simulink library "inp"  (R2021b)
settings: Solver=VariableStepAuto  StartTime=0.0  StopTime=10.0  RelTol=1e-3
undefined symbols (not defined in the file): C_TASK_5MS_S, FALSE, KINP_AcoreReadyToSlp_flg_ovrdflg, KINP_AcoreReadyToSlp_flg_ovrdval, KINP_AllowMovThd_OTA_enum_ovrdflg, KINP_AllowMovThd_OTA_enum_ovrdval, KINP_APSAngleTarget_Deg_ovrdflg, KINP_APSAngleTarget_Deg_ovrdval, KINP_APSDecReq_mps2_ovrdflg, KINP_APSDecReq_mps2_ovrdval, KINP_APSDecReqA_flg_ovrdflg, KINP_APSDecReqA_flg_ovrdval, KINP_APSDFLL_cm_ovrdflg, KINP_APSDFLL_cm_ovrdval, KINP_APSDFLR_cm_ovrdflg, KINP_APSDFLR_cm_ovrdval, KINP_APSDRLL_cm_ovrdflg, KINP_APSDRLL_cm_ovrdval, KINP_APSDRLR_cm_ovrdflg, KINP_APSDRLR_cm_ovrdval, KINP_APSExitCondition_enum_ovrdflg, KINP_APSExitCondition_enum_ovrdval, KINP_APSHWVer_enum_ovrdflg, KINP_APSHWVer_enum_ovrdval, KINP_APSProgressPCT_pct_ovrdflg, KINP_APSProgressPCT_pct_ovrdval, KINP_APSReq_enum_ovrdflg, KINP_APSReq_enum_ovrdval, KINP_APSRQDisplay_enum_ovrdflg, KINP_APSRQDisplay_enum_ovrdval, KINP_APSRqEPASCtrl_flg_ovrdflg, KINP_APSRqEPASCtrl_flg_ovrdval, KINP_APSShiftPosnReq_enum_ovrdval, KINP_APSShiftPosnReq_enum_ovrflg, KINP_APSSpeedCMD_kph_ovrdval, KINP_APSSpeedCMD_kph_ovrflg, KINP_APSStaSystem_enum_ovrdflg, KINP_APSStaSystem_enum_ovrdval, KINP_APSSWVer_enum_ovrdflg, KINP_APSSWVer_enum_ovrdval, KINP_APSVMCReqA_flg_ovrdval, KINP_APSVMCReqA_flg_ovrflg, KINP_APSVRqEPASCtrl_flg_ovrdflg, KINP_APSVRqEPASCtrl_flg_ovrdval, KINP_AuxBattVolmV_mV_ovrdflg, KINP_AuxBattVolmV_mV_ovrdval, KINP_CAASSta_enum_ovrdflg, KINP_CAASSta_enum_ovrdval, KINP_CAASVMCReqA_flg_ovrdval, KINP_CAASVMCReqA_flg_ovrflg, KINP_Chime_enum_ovrdflg, KINP_Chime_enum_ovrdval, KINP_ClearDTCcmd_flg_ovrdflg, KINP_ClearDTCcmd_flg_ovrdval, KINP_EvccAplusPwrUpReq_flg_ovrdflg, KINP_EvccAplusPwrUpReq_flg_ovrdval, KINP_LFID_raw_ovrdval, KINP_LFID_raw_ovrflg, KINP_LRID_raw_ovrdval, KINP_MemOffsetAccX_raw16_ovrdflg ... (+118)
libraries: FVT_lib x595, hcu_lib x1
(part 7 of 27)

== system inp/INP/CAN4/CreateBus ==
  inp_CanValid_bus : Inport
  inp_Hal_bus : Inport  Port=2
  UnitConverter_{1..14,24,26,31,34,38..40,44..49,60..61,63..64,97..99,102,108} (36 alike) : DataTypeConversion  OutDataTypeStr=boolean
  UnitConverter_{42..43,50..53,55..59,62,66,69,71,73,75,77,79,81,83,85,87,89..90,92..93,100..101,103..104,106,112,114,121,123,125,127,129,131,133,135,141} (43 alike) : DataTypeConversion  OutDataTypeStr=single
  UnitConverter_{15..23,25,30,32..33,35..37,41,54,65,67..68,70,72,74,76,78,80,82,84,86,88,91,94..96,105,107,109..111,113,115..120,122,124,126,128,130,132,134,136..140,142} (60 alike) : DataTypeConversion  OutDataTypeStr=uint8
  UnitConverter_27 : DataTypeConversion  OutDataTypeStr=uint64
  UnitConverter_28 : DataTypeConversion  OutDataTypeStr=uint64
  UnitConverter_29 : DataTypeConversion  OutDataTypeStr=uint64
  bus_creator : BusCreator  Inputs=142
  bus_selector : BusSelector  OutputSignals=VINP_CANMsgValidDKC1_flg,VINP_CANMsgValidDKC2_flg,VINP_CANMsgValidGWZDRPTG1_flg,VINP_CANMsgValidGWZoneDR1_flg,VINP_CANMsgValidGWZoneDR2_flg,VINP_CANMsgValidGWZoneDR3_flg,VINP_CANMsgValidGWZoneDR4_flg,VINP_CANMsgValidGWZoneDR6_flg,VINP_CANMsgValidGWZoneFR1_flg,VINP_CANMsgValidGWZoneFR2_flg,VINP_CANMsgValidZoneDrSCP_flg,VINP_CANMsgValidZoneDrTHCM_flg,VINP_CANMsgValidZoneDrVCU_flg,VINP_CANMsgValidZoneFrTHCM_flg
  bus_selector_1 : BusSelector  OutputSignals=VINP_DKCReVehData_enum,VINP_DKCRemotePW_enum,VINP_PCommandToBCM_enum,VINP_PCommandToPTG_enum,VINP_PDKeyAreaLockUnlock_enum,VINP_PDKeyAreaPS_enum,VINP_PDKeyAreaPTG_enum,VINP_PDKeyWelcome_enum,VINP_PDkeyShowIVI_enum,VINP_PKeyMiss_flg,VINP_PKeyMode_enum,VINP_PUIDLowPower_flg,VINP_EncryptionDATA063_enum,VINP_EncryptionDATA64127_enum,VINP_RandomNumberX_enum,VINP_PTGRDILSta_enum,VINP_CSWDimSw_flg,VINP_CSWFWasSwSta_enum,VINP_CSWFWipSwSta_enum,VINP_CSWPassSWSta_flg,VINP_CSWRWasSWSta_enum,VINP_CSWRWipIntSwSta_enum,VINP_CSWTurnSwSta_enum,VINP_DrLockSta_flg,VINP_MIRRORFOLDSW_flg,VINP_RLSLampSta_flg,VINP_RLSRainSnrWiperCmd_enum,VINP_RLTurnLampC_mA,VINP_RRTurnLampC_mA,VINP_RWiperAS_flg,VINP_RWiperProtection_flg,VINP_SWCCANCELSta_flg,VINP_SWCResUpSta_flg,VINP_SWCSetdownSta_flg,VINP_SWCmodeSta_flg,VINP_LDrvValWdwOpened_pct,VINP_LPasValWdwOpened_pct,VINP_LRLDValWdwOpened_pct,VINP_LRRDValWdwOpened_pct,VINP_PTGInnerSW2_enum,VINP_FrntPTCRearLeActHeatPwr_W,VINP_FrntPTCRearRiActHeatPwr_W,VINP_FrntPTCRiActHeatPwr_W,VINP_FLTurnLampC_mA,VINP_FRTurnLampC_mA,VINP_FWiperAS_flg,VINP_FWiperProtection_flg,VINP_COMPStatorSpd_rpm,VINP_CompProEN_flg,VINP_DrSCPSysErrLmp_flg,VINP_RegenMode_enum,VINP_SetSpd_kph,VINP_ZoneSpdCtrlMode_enum,VINP_BlowerErr_enum,VINP_SolarL_W,VINP_SolarLErr_enum,VINP_SolarR_W,VINP_SolarRErr_enum,VINP_TFaceL_C,VINP_TFaceLErr_enum,VINP_TFaceR_C,VINP_TFaceRErr_enum,VINP_TFaceRr_C,VINP_TFaceRrErr_enum,VINP_TFootL_C,VINP_TFootLErr_enum,VINP_TFootR_C,VINP_TFootRErr_enum,VINP_TFootRr_C,VINP_TFootRrErr_enum,VINP_Tevap_C,VINP_TevapErr_enum,VINP_Tincar_C,VINP_TincarErr_enum,VINP_DrAuBoxPwrN1Curr_A,VINP_DrAuBoxPwrN2Curr_A,VINP_DrColumnSWFault_enum,VINP_DrCtrlBDVolt_V,VINP_DrCtrlTemp_C,VINP_DrEOBDFault_enum,VINP_DrIVIFault_enum,VINP_DrInfoFault_enum,VINP_DrPMMLVOutPErrLmp_flg,VINP_DrPMMLimpHomeActReq_flg,VINP_DrPMMSysErrLmp_flg,VINP_DrPowerTemp1_C,VINP_DrPowerTemp2_C,VINP_DrPwrInformationSta_flg,VINP_DrPwrONA1Curr_A,VINP_DrPwrONA2Curr_A,VINP_DrPwrSta_enum,VINP_DrPwrStdbyACurr_A,VINP_DrPwrWindowECUFault_enum,VINP_DrStdAErrSta_flg,VINP_DrTHCMFault_enum,VINP_ZoneDrMalfunLevel_enum,VINP_AGSErr_enum,VINP_BatInTemp_C,VINP_BatInTempErr_enum,VINP_BatOutTemp_C,VINP_COMPErr_enum,VINP_EACProtectEnable_enum,VINP_EWP3Err_enum,VINP_EXV1Err_enum,VINP_EXV2Err_enum,VINP_FanErr_enum,VINP_MotorInTemp_C,VINP_MotorInTempErr_enum,VINP_MotorOutTemp_C,VINP_MotorOutTempErr_enum,VINP_PTHighP_KPa,VINP_PTHighPErr_enum,VINP_PTHighTact_C,VINP_PTHighTactErr_enum,VINP_PTLowP1_KPa,VINP_PTLowP1Err_enum,VINP_PTLowP2_KPa,VINP_PTLowP2Err_enum,VINP_PTLowT1_C,VINP_PTLowT1Err_enum,VINP_PTLowT2_C,VINP_PTLowT2Err_enum,VINP_SOTXVErr_enum,VINP_SOV1Err_enum,VINP_SOV2Err_enum,VINP_SOV3Err_enum,VINP_Tamb_C,VINP_TambErr_enum
  BINP_outputs : Outport
  wires:
  inp_CanValid_bus/1 -> [inp_CanValid_bus]
  inp_Hal_bus/1 -> [inp_Hal_bus]
  bus_selector/1 -> UnitConverter_1/1  "<VINP_CANMsgValidDKC1_flg>"
  UnitConverter_1/1 -> bus_creator/1  "VINP_CANMsgValidDKC1_flg"
  bus_selector/2 -> UnitConverter_2/1  "<VINP_CANMsgValidDKC2_flg>"
  UnitConverter_2/1 -> bus_creator/2  "VINP_CANMsgValidDKC2_flg"
  bus_selector/3 -> UnitConverter_3/1  "<VINP_CANMsgValidGWZDRPTG1_flg>"
  UnitConverter_3/1 -> bus_creator/3  "VINP_CANMsgValidGWZDRPTG1_flg"
  bus_selector/4 -> UnitConverter_4/1  "<VINP_CANMsgValidGWZoneDR1_flg>"
  UnitConverter_4/1 -> bus_creator/4  "VINP_CANMsgValidGWZoneDR1_flg"
  bus_selector/5 -> UnitConverter_5/1  "<VINP_CANMsgValidGWZoneDR2_flg>"
  UnitConverter_5/1 -> bus_creator/5  "VINP_CANMsgValidGWZoneDR2_flg"
  bus_selector/6 -> UnitConverter_6/1  "<VINP_CANMsgValidGWZoneDR3_flg>"
  UnitConverter_6/1 -> bus_creator/6  "VINP_CANMsgValidGWZoneDR3_flg"
  bus_selector/7 -> UnitConverter_7/1  "<VINP_CANMsgValidGWZoneDR4_flg>"
  UnitConverter_7/1 -> bus_creator/7  "VINP_CANMsgValidGWZoneDR4_flg"
  bus_selector/8 -> UnitConverter_8/1  "<VINP_CANMsgValidGWZoneDR6_flg>"
  UnitConverter_8/1 -> bus_creator/8  "VINP_CANMsgValidGWZoneDR6_flg"
  bus_selector/9 -> UnitConverter_9/1  "<VINP_CANMsgValidGWZoneFR1_flg>"
  UnitConverter_9/1 -> bus_creator/9  "VINP_CANMsgValidGWZoneFR1_flg"
  bus_selector/10 -> UnitConverter_10/1  "<VINP_CANMsgValidGWZoneFR2_flg>"
  UnitConverter_10/1 -> bus_creator/10  "VINP_CANMsgValidGWZoneFR2_flg"
  bus_selector/11 -> UnitConverter_11/1  "<VINP_CANMsgValidZoneDrSCP_flg>"
  UnitConverter_11/1 -> bus_creator/11  "VINP_CANMsgValidZoneDrSCP_flg"
  bus_selector/12 -> UnitConverter_12/1  "<VINP_CANMsgValidZoneDrTHCM_flg>"
  UnitConverter_12/1 -> bus_creator/12  "VINP_CANMsgValidZoneDrTHCM_flg"
  bus_selector/13 -> UnitConverter_13/1  "<VINP_CANMsgValidZoneDrVCU_flg>"
  UnitConverter_13/1 -> bus_creator/13  "VINP_CANMsgValidZoneDrVCU_flg"
  bus_selector/14 -> UnitConverter_14/1  "<VINP_CANMsgValidZoneFrTHCM_flg>"
  UnitConverter_14/1 -> bus_creator/14  "VINP_CANMsgValidZoneFrTHCM_flg"
  bus_selector_1/1 -> UnitConverter_15/1  "<VINP_DKCReVehData_enum>"
  UnitConverter_15/1 -> bus_creator/15  "VINP_DKCReVehData_enum"
  bus_selector_1/2 -> UnitConverter_16/1  "<VINP_DKCRemotePW_enum>"
  UnitConverter_16/1 -> bus_creator/16  "VINP_DKCRemotePW_enum"
  bus_selector_1/3 -> UnitConverter_17/1  "<VINP_PCommandToBCM_enum>"
  UnitConverter_17/1 -> bus_creator/17  "VINP_PCommandToBCM_enum"
  bus_selector_1/4 -> UnitConverter_18/1  "<VINP_PCommandToPTG_enum>"
  UnitConverter_18/1 -> bus_creator/18  "VINP_PCommandToPTG_enum"
  bus_selector_1/5 -> UnitConverter_19/1  "<VINP_PDKeyAreaLockUnlock_enum>"
  UnitConverter_19/1 -> bus_creator/19  "VINP_PDKeyAreaLockUnlock_enum"
  bus_selector_1/6 -> UnitConverter_20/1  "<VINP_PDKeyAreaPS_enum>"
  UnitConverter_20/1 -> bus_creator/20  "VINP_PDKeyAreaPS_enum"
  bus_selector_1/7 -> UnitConverter_21/1  "<VINP_PDKeyAreaPTG_enum>"
  UnitConverter_21/1 -> bus_creator/21  "VINP_PDKeyAreaPTG_enum"
  bus_selector_1/8 -> UnitConverter_22/1  "<VINP_PDKeyWelcome_enum>"
  UnitConverter_22/1 -> bus_creator/22  "VINP_PDKeyWelcome_enum"
  bus_selector_1/9 -> UnitConverter_23/1  "<VINP_PDkeyShowIVI_enum>"
  UnitConverter_23/1 -> bus_creator/23  "VINP_PDkeyShowIVI_enum"
  bus_selector_1/10 -> UnitConverter_24/1  "<VINP_PKeyMiss_flg>"
  UnitConverter_24/1 -> bus_creator/24  "VINP_PKeyMiss_flg"
  bus_selector_1/11 -> UnitConverter_25/1  "<VINP_PKeyMode_enum>"
  UnitConverter_25/1 -> bus_creator/25  "VINP_PKeyMode_enum"
  bus_selector_1/12 -> UnitConverter_26/1  "<VINP_PUIDLowPower_flg>"
  UnitConverter_26/1 -> bus_creator/26  "VINP_PUIDLowPower_flg"
  bus_selector_1/13 -> UnitConverter_27/1  "<VINP_EncryptionDATA063_enum>"
  UnitConverter_27/1 -> bus_creator/27  "VINP_EncryptionDATA063_enum"
  bus_selector_1/14 -> UnitConverter_28/1  "<VINP_EncryptionDATA64127_enum>"
  UnitConverter_28/1 -> bus_creator/28  "VINP_EncryptionDATA64127_enum"
  bus_selector_1/15 -> UnitConverter_29/1  "<VINP_RandomNumberX_enum>"
  UnitConverter_29/1 -> bus_creator/29  "VINP_RandomNumberX_enum"
  bus_selector_1/16 -> UnitConverter_30/1  "<VINP_PTGRDILSta_enum>"
  UnitConverter_30/1 -> bus_creator/30  "VINP_PTGRDILSta_enum"
  bus_selector_1/17 -> UnitConverter_31/1  "<VINP_CSWDimSw_flg>"
  UnitConverter_31/1 -> bus_creator/31  "VINP_CSWDimSw_flg"
  bus_selector_1/18 -> UnitConverter_32/1  "<VINP_CSWFWasSwSta_enum>"
  UnitConverter_32/1 -> bus_creator/32  "VINP_CSWFWasSwSta_enum"
  bus_selector_1/19 -> UnitConverter_33/1  "<VINP_CSWFWipSwSta_enum>"
  UnitConverter_33/1 -> bus_creator/33  "VINP_CSWFWipSwSta_enum"
  bus_selector_1/20 -> UnitConverter_34/1  "<VINP_CSWPassSWSta_flg>"
  UnitConverter_34/1 -> bus_creator/34  "VINP_CSWPassSWSta_flg"
  bus_selector_1/21 -> UnitConverter_35/1  "<VINP_CSWRWasSWSta_enum>"
  UnitConverter_35/1 -> bus_creator/35  "VINP_CSWRWasSWSta_enum"
  bus_selector_1/22 -> UnitConverter_36/1  "<VINP_CSWRWipIntSwSta_enum>"
  UnitConverter_36/1 -> bus_creator/36  "VINP_CSWRWipIntSwSta_enum"
  bus_selector_1/23 -> UnitConverter_37/1  "<VINP_CSWTurnSwSta_enum>"
  UnitConverter_37/1 -> bus_creator/37  "VINP_CSWTurnSwSta_enum"
  bus_selector_1/24 -> UnitConverter_38/1  "<VINP_DrLockSta_flg>"
  UnitConverter_38/1 -> bus_creator/38  "VINP_DrLockSta_flg"
  bus_selector_1/25 -> UnitConverter_39/1  "<VINP_MIRRORFOLDSW_flg>"
  UnitConverter_39/1 -> bus_creator/39  "VINP_MIRRORFOLDSW_flg"
  bus_selector_1/26 -> UnitConverter_40/1  "<VINP_RLSLampSta_flg>"
  UnitConverter_40/1 -> bus_creator/40  "VINP_RLSLampSta_flg"
  bus_selector_1/27 -> UnitConverter_41/1  "<VINP_RLSRainSnrWiperCmd_enum>"
  UnitConverter_41/1 -> bus_creator/41  "VINP_RLSRainSnrWiperCmd_enum"
  bus_selector_1/28 -> UnitConverter_42/1  "<VINP_RLTurnLampC_mA>"
  UnitConverter_42/1 -> bus_creator/42  "VINP_RLTurnLampC_mA"
  bus_selector_1/29 -> UnitConverter_43/1  "<VINP_RRTurnLampC_mA>"
  UnitConverter_43/1 -> bus_creator/43  "VINP_RRTurnLampC_mA"
  bus_selector_1/30 -> UnitConverter_44/1  "<VINP_RWiperAS_flg>"
  UnitConverter_44/1 -> bus_creator/44  "VINP_RWiperAS_flg"
  bus_selector_1/31 -> UnitConverter_45/1  "<VINP_RWiperProtection_flg>"
  UnitConverter_45/1 -> bus_creator/45  "VINP_RWiperProtection_flg"
  bus_selector_1/32 -> UnitConverter_46/1  "<VINP_SWCCANCELSta_flg>"
  UnitConverter_46/1 -> bus_creator/46  "VINP_SWCCANCELSta_flg"
  bus_selector_1/33 -> UnitConverter_47/1  "<VINP_SWCResUpSta_flg>"
  UnitConverter_47/1 -> bus_creator/47  "VINP_SWCResUpSta_flg"
  bus_selector_1/34 -> UnitConverter_48/1  "<VINP_SWCSetdownSta_flg>"
  UnitConverter_48/1 -> bus_creator/48  "VINP_SWCSetdownSta_flg"
  bus_selector_1/35 -> UnitConverter_49/1  "<VINP_SWCmodeSta_flg>"
  UnitConverter_49/1 -> bus_creator/49  "VINP_SWCmodeSta_flg"
  bus_selector_1/36 -> UnitConverter_50/1  "<VINP_LDrvValWdwOpened_pct>"
  UnitConverter_50/1 -> bus_creator/50  "VINP_LDrvValWdwOpened_pct"
  bus_selector_1/37 -> UnitConverter_51/1  "<VINP_LPasValWdwOpened_pct>"
  UnitConverter_51/1 -> bus_creator/51  "VINP_LPasValWdwOpened_pct"
  bus_selector_1/38 -> UnitConverter_52/1  "<VINP_LRLDValWdwOpened_pct>"
  UnitConverter_52/1 -> bus_creator/52  "VINP_LRLDValWdwOpened_pct"
  bus_selector_1/39 -> UnitConverter_53/1  "<VINP_LRRDValWdwOpened_pct>"
  UnitConverter_53/1 -> bus_creator/53  "VINP_LRRDValWdwOpened_pct"
  bus_selector_1/40 -> UnitConverter_54/1  "<VINP_PTGInnerSW2_enum>"
  UnitConverter_54/1 -> bus_creator/54  "VINP_PTGInnerSW2_enum"
  bus_selector_1/41 -> UnitConverter_55/1  "<VINP_FrntPTCRearLeActHeatPwr_W>"
  UnitConverter_55/1 -> bus_creator/55  "VINP_FrntPTCRearLeActHeatPwr_W"
  bus_selector_1/42 -> UnitConverter_56/1  "<VINP_FrntPTCRearRiActHeatPwr_W>"
  UnitConverter_56/1 -> bus_creator/56  "VINP_FrntPTCRearRiActHeatPwr_W"
  bus_selector_1/43 -> UnitConverter_57/1  "<VINP_FrntPTCRiActHeatPwr_W>"
  UnitConverter_57/1 -> bus_creator/57  "VINP_FrntPTCRiActHeatPwr_W"
  bus_selector_1/44 -> UnitConverter_58/1  "<VINP_FLTurnLampC_mA>"
  UnitConverter_58/1 -> bus_creator/58  "VINP_FLTurnLampC_mA"
  bus_selector_1/45 -> UnitConverter_59/1  "<VINP_FRTurnLampC_mA>"
  UnitConverter_59/1 -> bus_creator/59  "VINP_FRTurnLampC_mA"
  bus_selector_1/46 -> UnitConverter_60/1  "<VINP_FWiperAS_flg>"
  UnitConverter_60/1 -> bus_creator/60  "VINP_FWiperAS_flg"
  bus_selector_1/47 -> UnitConverter_61/1  "<VINP_FWiperProtection_flg>"
  UnitConverter_61/1 -> bus_creator/61  "VINP_FWiperProtection_flg"
  bus_selector_1/48 -> UnitConverter_62/1  "<VINP_COMPStatorSpd_rpm>"
  UnitConverter_62/1 -> bus_creator/62  "VINP_COMPStatorSpd_rpm"
  bus_selector_1/49 -> UnitConverter_63/1  "<VINP_CompProEN_flg>"
  UnitConverter_63/1 -> bus_creator/63  "VINP_CompProEN_flg"
  bus_selector_1/50 -> UnitConverter_64/1  "<VINP_DrSCPSysErrLmp_flg>"
  UnitConverter_64/1 -> bus_creator/64  "VINP_DrSCPSysErrLmp_flg"
  bus_selector_1/51 -> UnitConverter_65/1  "<VINP_RegenMode_enum>"
  UnitConverter_65/1 -> bus_creator/65  "VINP_RegenMode_enum"
  bus_selector_1/52 -> UnitConverter_66/1  "<VINP_SetSpd_kph>"
  UnitConverter_66/1 -> bus_creator/66  "VINP_SetSpd_kph"
  bus_selector_1/53 -> UnitConverter_67/1  "<VINP_ZoneSpdCtrlMode_enum>"
  UnitConverter_67/1 -> bus_creator/67  "VINP_ZoneSpdCtrlMode_enum"
  bus_selector_1/54 -> UnitConverter_68/1  "<VINP_BlowerErr_enum>"
  UnitConverter_68/1 -> bus_creator/68  "VINP_BlowerErr_enum"
  bus_selector_1/55 -> UnitConverter_69/1  "<VINP_SolarL_W>"
  UnitConverter_69/1 -> bus_creator/69  "VINP_SolarL_W"
  bus_selector_1/56 -> UnitConverter_70/1  "<VINP_SolarLErr_enum>"
  UnitConverter_70/1 -> bus_creator/70  "VINP_SolarLErr_enum"
  bus_selector_1/57 -> UnitConverter_71/1  "<VINP_SolarR_W>"
  UnitConverter_71/1 -> bus_creator/71  "VINP_SolarR_W"
  bus_selector_1/58 -> UnitConverter_72/1  "<VINP_SolarRErr_enum>"
  UnitConverter_72/1 -> bus_creator/72  "VINP_SolarRErr_enum"
  bus_selector_1/59 -> UnitConverter_73/1  "<VINP_TFaceL_C>"
  UnitConverter_73/1 -> bus_creator/73  "VINP_TFaceL_C"
  bus_selector_1/60 -> UnitConverter_74/1  "<VINP_TFaceLErr_enum>"
  UnitConverter_74/1 -> bus_creator/74  "VINP_TFaceLErr_enum"
  bus_selector_1/61 -> UnitConverter_75/1  "<VINP_TFaceR_C>"
  UnitConverter_75/1 -> bus_creator/75  "VINP_TFaceR_C"
  bus_selector_1/62 -> UnitConverter_76/1  "<VINP_TFaceRErr_enum>"
  UnitConverter_76/1 -> bus_creator/76  "VINP_TFaceRErr_enum"
  bus_selector_1/63 -> UnitConverter_77/1  "<VINP_TFaceRr_C>"
  UnitConverter_77/1 -> bus_creator/77  "VINP_TFaceRr_C"
  bus_selector_1/64 -> UnitConverter_78/1  "<VINP_TFaceRrErr_enum>"
  UnitConverter_78/1 -> bus_creator/78  "VINP_TFaceRrErr_enum"
  bus_selector_1/65 -> UnitConverter_79/1  "<VINP_TFootL_C>"
  UnitConverter_79/1 -> bus_creator/79  "VINP_TFootL_C"
  bus_selector_1/66 -> UnitConverter_80/1  "<VINP_TFootLErr_enum>"
  UnitConverter_80/1 -> bus_creator/80  "VINP_TFootLErr_enum"
  bus_selector_1/67 -> UnitConverter_81/1  "<VINP_TFootR_C>"
  UnitConverter_81/1 -> bus_creator/81  "VINP_TFootR_C"
  bus_selector_1/68 -> UnitConverter_82/1  "<VINP_TFootRErr_enum>"
  UnitConverter_82/1 -> bus_creator/82  "VINP_TFootRErr_enum"
  bus_selector_1/69 -> UnitConverter_83/1  "<VINP_TFootRr_C>"
  UnitConverter_83/1 -> bus_creator/83  "VINP_TFootRr_C"
  bus_selector_1/70 -> UnitConverter_84/1  "<VINP_TFootRrErr_enum>"
  UnitConverter_84/1 -> bus_creator/84  "VINP_TFootRrErr_enum"
  bus_selector_1/71 -> UnitConverter_85/1  "<VINP_Tevap_C>"
  UnitConverter_85/1 -> bus_creator/85  "VINP_Tevap_C"
  bus_selector_1/72 -> UnitConverter_86/1  "<VINP_TevapErr_enum>"
  UnitConverter_86/1 -> bus_creator/86  "VINP_TevapErr_enum"
  bus_selector_1/73 -> UnitConverter_87/1  "<VINP_Tincar_C>"
  UnitConverter_87/1 -> bus_creator/87  "VINP_Tincar_C"
  bus_selector_1/74 -> UnitConverter_88/1  "<VINP_TincarErr_enum>"
  UnitConverter_88/1 -> bus_creator/88  "VINP_TincarErr_enum"
  bus_selector_1/75 -> UnitConverter_89/1  "<VINP_DrAuBoxPwrN1Curr_A>"
  UnitConverter_89/1 -> bus_creator/89  "VINP_DrAuBoxPwrN1Curr_A"
  bus_selector_1/76 -> UnitConverter_90/1  "<VINP_DrAuBoxPwrN2Curr_A>"
  UnitConverter_90/1 -> bus_creator/90  "VINP_DrAuBoxPwrN2Curr_A"
  bus_selector_1/77 -> UnitConverter_91/1  "<VINP_DrColumnSWFault_enum>"
  UnitConverter_91/1 -> bus_creator/91  "VINP_DrColumnSWFault_enum"
  bus_selector_1/78 -> UnitConverter_92/1  "<VINP_DrCtrlBDVolt_V>"
  UnitConverter_92/1 -> bus_creator/92  "VINP_DrCtrlBDVolt_V"
  bus_selector_1/79 -> UnitConverter_93/1  "<VINP_DrCtrlTemp_C>"
  UnitConverter_93/1 -> bus_creator/93  "VINP_DrCtrlTemp_C"
  bus_selector_1/80 -> UnitConverter_94/1  "<VINP_DrEOBDFault_enum>"
  UnitConverter_94/1 -> bus_creator/94  "VINP_DrEOBDFault_enum"
  bus_selector_1/81 -> UnitConverter_95/1  "<VINP_DrIVIFault_enum>"
  UnitConverter_95/1 -> bus_creator/95  "VINP_DrIVIFault_enum"
  bus_selector_1/82 -> UnitConverter_96/1  "<VINP_DrInfoFault_enum>"
  UnitConverter_96/1 -> bus_creator/96  "VINP_DrInfoFault_enum"
  bus_selector_1/83 -> UnitConverter_97/1  "<VINP_DrPMMLVOutPErrLmp_flg>"
  UnitConverter_97/1 -> bus_creator/97  "VINP_DrPMMLVOutPErrLmp_flg"
  bus_selector_1/84 -> UnitConverter_98/1  "<VINP_DrPMMLimpHomeActReq_flg>"
  UnitConverter_98/1 -> bus_creator/98  "VINP_DrPMMLimpHomeActReq_flg"
  bus_selector_1/85 -> UnitConverter_99/1  "<VINP_DrPMMSysErrLmp_flg>"
  UnitConverter_99/1 -> bus_creator/99  "VINP_DrPMMSysErrLmp_flg"
  bus_selector_1/86 -> UnitConverter_100/1  "<VINP_DrPowerTemp1_C>"
  UnitConverter_100/1 -> bus_creator/100  "VINP_DrPowerTemp1_C"
  bus_selector_1/87 -> UnitConverter_101/1  "<VINP_DrPowerTemp2_C>"
  UnitConverter_101/1 -> bus_creator/101  "VINP_DrPowerTemp2_C"
  bus_selector_1/88 -> UnitConverter_102/1  "<VINP_DrPwrInformationSta_flg>"
  UnitConverter_102/1 -> bus_creator/102  "VINP_DrPwrInformationSta_flg"
  bus_selector_1/89 -> UnitConverter_103/1  "<VINP_DrPwrONA1Curr_A>"
  UnitConverter_103/1 -> bus_creator/103  "VINP_DrPwrONA1Curr_A"
  bus_selector_1/90 -> UnitConverter_104/1  "<VINP_DrPwrONA2Curr_A>"
  UnitConverter_104/1 -> bus_creator/104  "VINP_DrPwrONA2Curr_A"
  bus_selector_1/91 -> UnitConverter_105/1  "<VINP_DrPwrSta_enum>"
  UnitConverter_105/1 -> bus_creator/105  "VINP_DrPwrSta_enum"
  bus_selector_1/92 -> UnitConverter_106/1  "<VINP_DrPwrStdbyACurr_A>"
  UnitConverter_106/1 -> bus_creator/106  "VINP_DrPwrStdbyACurr_A"
  bus_selector_1/93 -> UnitConverter_107/1  "<VINP_DrPwrWindowECUFault_enum>"
  UnitConverter_107/1 -> bus_creator/107  "VINP_DrPwrWindowECUFault_enum"
  bus_selector_1/94 -> UnitConverter_108/1  "<VINP_DrStdAErrSta_flg>"
  UnitConverter_108/1 -> bus_creator/108  "VINP_DrStdAErrSta_flg"
  bus_selector_1/95 -> UnitConverter_109/1  "<VINP_DrTHCMFault_enum>"
  UnitConverter_109/1 -> bus_creator/109  "VINP_DrTHCMFault_enum"
  bus_selector_1/96 -> UnitConverter_110/1  "<VINP_ZoneDrMalfunLevel_enum>"
  UnitConverter_110/1 -> bus_creator/110  "VINP_ZoneDrMalfunLevel_enum"
  bus_selector_1/97 -> UnitConverter_111/1  "<VINP_AGSErr_enum>"
  UnitConverter_111/1 -> bus_creator/111  "VINP_AGSErr_enum"
  bus_selector_1/98 -> UnitConverter_112/1  "<VINP_BatInTemp_C>"
  UnitConverter_112/1 -> bus_creator/112  "VINP_BatInTemp_C"
  bus_selector_1/99 -> UnitConverter_113/1  "<VINP_BatInTempErr_enum>"
  UnitConverter_113/1 -> bus_creator/113  "VINP_BatInTempErr_enum"
  bus_selector_1/100 -> UnitConverter_114/1  "<VINP_BatOutTemp_C>"
  UnitConverter_114/1 -> bus_creator/114  "VINP_BatOutTemp_C"
  bus_selector_1/101 -> UnitConverter_115/1  "<VINP_COMPErr_enum>"
  UnitConverter_115/1 -> bus_creator/115  "VINP_COMPErr_enum"
  bus_selector_1/102 -> UnitConverter_116/1  "<VINP_EACProtectEnable_enum>"
  UnitConverter_116/1 -> bus_creator/116  "VINP_EACProtectEnable_enum"
  bus_selector_1/103 -> UnitConverter_117/1  "<VINP_EWP3Err_enum>"
  UnitConverter_117/1 -> bus_creator/117  "VINP_EWP3Err_enum"
  bus_selector_1/104 -> UnitConverter_118/1  "<VINP_EXV1Err_enum>"
  UnitConverter_118/1 -> bus_creator/118  "VINP_EXV1Err_enum"
  bus_selector_1/105 -> UnitConverter_119/1  "<VINP_EXV2Err_enum>"
  UnitConverter_119/1 -> bus_creator/119  "VINP_EXV2Err_enum"
  bus_selector_1/106 -> UnitConverter_120/1  "<VINP_FanErr_enum>"
  UnitConverter_120/1 -> bus_creator/120  "VINP_FanErr_enum"
  bus_selector_1/107 -> UnitConverter_121/1  "<VINP_MotorInTemp_C>"
  UnitConverter_121/1 -> bus_creator/121  "VINP_MotorInTemp_C"
  bus_selector_1/108 -> UnitConverter_122/1  "<VINP_MotorInTempErr_enum>"
  UnitConverter_122/1 -> bus_creator/122  "VINP_MotorInTempErr_enum"
  bus_selector_1/109 -> UnitConverter_123/1  "<VINP_MotorOutTemp_C>"
  UnitConverter_123/1 -> bus_creator/123  "VINP_MotorOutTemp_C"
  bus_selector_1/110 -> UnitConverter_124/1  "<VINP_MotorOutTempErr_enum>"
  UnitConverter_124/1 -> bus_creator/124  "VINP_MotorOutTempErr_enum"
  bus_selector_1/111 -> UnitConverter_125/1  "<VINP_PTHighP_KPa>"
  UnitConverter_125/1 -> bus_creator/125  "VINP_PTHighP_KPa"
  bus_selector_1/112 -> UnitConverter_126/1  "<VINP_PTHighPErr_enum>"
  UnitConverter_126/1 -> bus_creator/126  "VINP_PTHighPErr_enum"
  bus_selector_1/113 -> UnitConverter_127/1  "<VINP_PTHighTact_C>"
  UnitConverter_127/1 -> bus_creator/127  "VINP_PTHighTact_C"
  bus_selector_1/114 -> UnitConverter_128/1  "<VINP_PTHighTactErr_enum>"
  UnitConverter_128/1 -> bus_creator/128  "VINP_PTHighTactErr_enum"
  bus_selector_1/115 -> UnitConverter_129/1  "<VINP_PTLowP1_KPa>"
  UnitConverter_129/1 -> bus_creator/129  "VINP_PTLowP1_KPa"
  bus_selector_1/116 -> UnitConverter_130/1  "<VINP_PTLowP1Err_enum>"
  UnitConverter_130/1 -> bus_creator/130  "VINP_PTLowP1Err_enum"
  bus_selector_1/117 -> UnitConverter_131/1  "<VINP_PTLowP2_KPa>"
  UnitConverter_131/1 -> bus_creator/131  "VINP_PTLowP2_KPa"
  bus_selector_1/118 -> UnitConverter_132/1  "<VINP_PTLowP2Err_enum>"
  UnitConverter_132/1 -> bus_creator/132  "VINP_PTLowP2Err_enum"
  bus_selector_1/119 -> UnitConverter_133/1  "<VINP_PTLowT1_C>"
  UnitConverter_133/1 -> bus_creator/133  "VINP_PTLowT1_C"
  bus_selector_1/120 -> UnitConverter_134/1  "<VINP_PTLowT1Err_enum>"
  UnitConverter_134/1 -> bus_creator/134  "VINP_PTLowT1Err_enum"
  bus_selector_1/121 -> UnitConverter_135/1  "<VINP_PTLowT2_C>"
  UnitConverter_135/1 -> bus_creator/135  "VINP_PTLowT2_C"
  bus_selector_1/122 -> UnitConverter_136/1  "<VINP_PTLowT2Err_enum>"
  UnitConverter_136/1 -> bus_creator/136  "VINP_PTLowT2Err_enum"
  bus_selector_1/123 -> UnitConverter_137/1  "<VINP_SOTXVErr_enum>"
  UnitConverter_137/1 -> bus_creator/137  "VINP_SOTXVErr_enum"
  bus_selector_1/124 -> UnitConverter_138/1  "<VINP_SOV1Err_enum>"
  UnitConverter_138/1 -> bus_creator/138  "VINP_SOV1Err_enum"
  bus_selector_1/125 -> UnitConverter_139/1  "<VINP_SOV2Err_enum>"
  UnitConverter_139/1 -> bus_creator/139  "VINP_SOV2Err_enum"
  bus_selector_1/126 -> UnitConverter_140/1  "<VINP_SOV3Err_enum>"
  UnitConverter_140/1 -> bus_creator/140  "VINP_SOV3Err_enum"
  bus_selector_1/127 -> UnitConverter_141/1  "<VINP_Tamb_C>"
  UnitConverter_141/1 -> bus_creator/141  "VINP_Tamb_C"
  bus_selector_1/128 -> UnitConverter_142/1  "<VINP_TambErr_enum>"
  UnitConverter_142/1 -> bus_creator/142  "VINP_TambErr_enum"
  [inp_CanValid_bus] -> bus_selector/1
  [inp_Hal_bus] -> bus_selector_1/1
  bus_creator/1 -> BINP_outputs/1

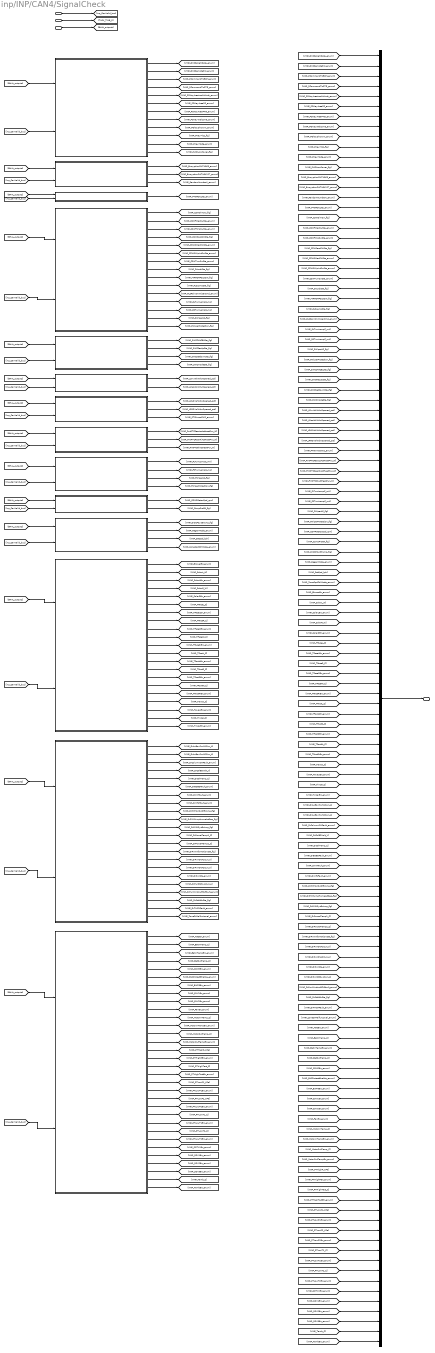
== system inp/INP/CAN4/SignalCheck ==
  inp_CanValid_bus : Inport
  TASK_TIME_S : Inport  Port=2
  BHAL_outputs : Inport  Port=3
  DKC1 : Subsystem
  DKC2 : Subsystem
  GW_ZDR_PTG1 : Subsystem
  GW_ZoneDR1 : Subsystem
  GW_ZoneDR2 : Subsystem
  GW_ZoneDR3 : Subsystem
  GW_ZoneDR4 : Subsystem
  GW_ZoneDR6 : Subsystem
  GW_ZoneFR1 : Subsystem
  GW_ZoneFR2 : Subsystem
  Zone_Dr_SCP : Subsystem
  Zone_Dr_THCM : Subsystem
  Zone_Dr_VCU : Subsystem
  Zone_Fr_THCM : Subsystem
  bus_creator : BusCreator  Inputs=128
  inp_Hal_bus : Outport
  wires:
  inp_CanValid_bus/1 -> [inp_CanValid_bus]
  TASK_TIME_S/1 -> [TASK_TIME_S]
  BHAL_outputs/1 -> [BHAL_outputs]
  [BHAL_outputs] -> DKC1/1(BHAL_outputs)
  [inp_CanValid_bus] -> DKC1/2(inp_CanValid_bus)
  DKC1/1(VINP_DKCReVehData_enum) -> [VINP_DKCReVehData_enum]
  DKC1/2(VINP_DKCRemotePW_enum) -> [VINP_DKCRemotePW_enum]
  DKC1/3(VINP_PCommandToBCM_enum) -> [VINP_PCommandToBCM_enum]
  DKC1/4(VINP_PCommandToPTG_enum) -> [VINP_PCommandToPTG_enum]
  DKC1/5(VINP_PDKeyAreaLockUnlock_enum) -> [VINP_PDKeyAreaLockUnlock_enum]
  DKC1/6(VINP_PDKeyAreaPS_enum) -> [VINP_PDKeyAreaPS_enum]
  DKC1/7(VINP_PDKeyAreaPTG_enum) -> [VINP_PDKeyAreaPTG_enum]
  DKC1/8(VINP_PDKeyWelcome_enum) -> [VINP_PDKeyWelcome_enum]
  DKC1/9(VINP_PDkeyShowIVI_enum) -> [VINP_PDkeyShowIVI_enum]
  DKC1/10(VINP_PKeyMiss_flg) -> [VINP_PKeyMiss_flg]
  DKC1/11(VINP_PKeyMode_enum) -> [VINP_PKeyMode_enum]
  DKC1/12(VINP_PUIDLowPower_flg) -> [VINP_PUIDLowPower_flg]
  [BHAL_outputs] -> DKC2/1(BHAL_outputs)
  [inp_CanValid_bus] -> DKC2/2(inp_CanValid_bus)
  DKC2/1(VINP_EncryptionDATA063_enum) -> [VINP_EncryptionDATA063_enum]
  DKC2/2(VINP_EncryptionDATA64127_enum) -> [VINP_EncryptionDATA64127_enum]
  DKC2/3(VINP_RandomNumberX_enum) -> [VINP_RandomNumberX_enum]
  [BHAL_outputs] -> GW_ZDR_PTG1/1(BHAL_outputs)
  [inp_CanValid_bus] -> GW_ZDR_PTG1/2(inp_CanValid_bus)
  GW_ZDR_PTG1/1(VINP_PTGRDILSta_enum) -> [VINP_PTGRDILSta_enum]
  [BHAL_outputs] -> GW_ZoneDR1/1(BHAL_outputs)
  [inp_CanValid_bus] -> GW_ZoneDR1/2(inp_CanValid_bus)
  GW_ZoneDR1/1(VINP_CSWDimSw_flg) -> [VINP_CSWDimSw_flg]
  GW_ZoneDR1/2(VINP_CSWFWasSwSta_enum) -> [VINP_CSWFWasSwSta_enum]
  GW_ZoneDR1/3(VINP_CSWFWipSwSta_enum) -> [VINP_CSWFWipSwSta_enum]
  GW_ZoneDR1/4(VINP_CSWPassSWSta_flg) -> [VINP_CSWPassSWSta_flg]
  GW_ZoneDR1/5(VINP_CSWRWasSWSta_enum) -> [VINP_CSWRWasSWSta_enum]
  GW_ZoneDR1/6(VINP_CSWRWipIntSwSta_enum) -> [VINP_CSWRWipIntSwSta_enum]
  GW_ZoneDR1/7(VINP_CSWTurnSwSta_enum) -> [VINP_CSWTurnSwSta_enum]
  GW_ZoneDR1/8(VINP_DrLockSta_flg) -> [VINP_DrLockSta_flg]
  GW_ZoneDR1/9(VINP_MIRRORFOLDSW_flg) -> [VINP_MIRRORFOLDSW_flg]
  GW_ZoneDR1/10(VINP_RLSLampSta_flg) -> [VINP_RLSLampSta_flg]
  GW_ZoneDR1/11(VINP_RLSRainSnrWiperCmd_enum) -> [VINP_RLSRainSnrWiperCmd_enum]
  GW_ZoneDR1/12(VINP_RLTurnLampC_mA) -> [VINP_RLTurnLampC_mA]
  GW_ZoneDR1/13(VINP_RRTurnLampC_mA) -> [VINP_RRTurnLampC_mA]
  GW_ZoneDR1/14(VINP_RWiperAS_flg) -> [VINP_RWiperAS_flg]
  GW_ZoneDR1/15(VINP_RWiperProtection_flg) -> [VINP_RWiperProtection_flg]
  [BHAL_outputs] -> GW_ZoneDR2/1(BHAL_outputs)
  [inp_CanValid_bus] -> GW_ZoneDR2/2(inp_CanValid_bus)
  GW_ZoneDR2/1(VINP_SWCCANCELSta_flg) -> [VINP_SWCCANCELSta_flg]
  GW_ZoneDR2/2(VINP_SWCResUpSta_flg) -> [VINP_SWCResUpSta_flg]
  GW_ZoneDR2/3(VINP_SWCSetdownSta_flg) -> [VINP_SWCSetdownSta_flg]
  GW_ZoneDR2/4(VINP_SWCmodeSta_flg) -> [VINP_SWCmodeSta_flg]
  [BHAL_outputs] -> GW_ZoneDR3/1(BHAL_outputs)
  [inp_CanValid_bus] -> GW_ZoneDR3/2(inp_CanValid_bus)
  GW_ZoneDR3/1(VINP_LDrvValWdwOpened_pct) -> [VINP_LDrvValWdwOpened_pct]
  GW_ZoneDR3/2(VINP_LPasValWdwOpened_pct) -> [VINP_LPasValWdwOpened_pct]
  [BHAL_outputs] -> GW_ZoneDR4/1(BHAL_outputs)
  [inp_CanValid_bus] -> GW_ZoneDR4/2(inp_CanValid_bus)
  GW_ZoneDR4/1(VINP_LRLDValWdwOpened_pct) -> [VINP_LRLDValWdwOpened_pct]
  GW_ZoneDR4/2(VINP_LRRDValWdwOpened_pct) -> [VINP_LRRDValWdwOpened_pct]
  GW_ZoneDR4/3(VINP_PTGInnerSW2_enum) -> [VINP_PTGInnerSW2_enum]
  [BHAL_outputs] -> GW_ZoneDR6/1(BHAL_outputs)
  [inp_CanValid_bus] -> GW_ZoneDR6/2(inp_CanValid_bus)
  GW_ZoneDR6/1(VINP_FrntPTCRearLeActHeatPwr_W) -> [VINP_FrntPTCRearLeActHeatPwr_W]
  GW_ZoneDR6/2(VINP_FrntPTCRearRiActHeatPwr_W) -> [VINP_FrntPTCRearRiActHeatPwr_W]
  GW_ZoneDR6/3(VINP_FrntPTCRiActHeatPwr_W) -> [VINP_FrntPTCRiActHeatPwr_W]
  [BHAL_outputs] -> GW_ZoneFR1/1(BHAL_outputs)
  [inp_CanValid_bus] -> GW_ZoneFR1/2(inp_CanValid_bus)
  GW_ZoneFR1/1(VINP_FLTurnLampC_mA) -> [VINP_FLTurnLampC_mA]
  GW_ZoneFR1/2(VINP_FRTurnLampC_mA) -> [VINP_FRTurnLampC_mA]
  GW_ZoneFR1/3(VINP_FWiperAS_flg) -> [VINP_FWiperAS_flg]
  GW_ZoneFR1/4(VINP_FWiperProtection_flg) -> [VINP_FWiperProtection_flg]
  [BHAL_outputs] -> GW_ZoneFR2/1(BHAL_outputs)
  [inp_CanValid_bus] -> GW_ZoneFR2/2(inp_CanValid_bus)
  GW_ZoneFR2/1(VINP_COMPStatorSpd_rpm) -> [VINP_COMPStatorSpd_rpm]
  GW_ZoneFR2/2(VINP_CompProEN_flg) -> [VINP_CompProEN_flg]
  [BHAL_outputs] -> Zone_Dr_SCP/1(BHAL_outputs)
  [inp_CanValid_bus] -> Zone_Dr_SCP/2(inp_CanValid_bus)
  Zone_Dr_SCP/1(VINP_DrSCPSysErrLmp_flg) -> [VINP_DrSCPSysErrLmp_flg]
  Zone_Dr_SCP/2(VINP_RegenMode_enum) -> [VINP_RegenMode_enum]
  Zone_Dr_SCP/3(VINP_SetSpd_kph) -> [VINP_SetSpd_kph]
  Zone_Dr_SCP/4(VINP_ZoneSpdCtrlMode_enum) -> [VINP_ZoneSpdCtrlMode_enum]
  [BHAL_outputs] -> Zone_Dr_THCM/1(BHAL_outputs)
  [inp_CanValid_bus] -> Zone_Dr_THCM/2(inp_CanValid_bus)
  Zone_Dr_THCM/1(VINP_BlowerErr_enum) -> [VINP_BlowerErr_enum]
  Zone_Dr_THCM/2(VINP_SolarL_W) -> [VINP_SolarL_W]
  Zone_Dr_THCM/3(VINP_SolarLErr_enum) -> [VINP_SolarLErr_enum]
  Zone_Dr_THCM/4(VINP_SolarR_W) -> [VINP_SolarR_W]
  Zone_Dr_THCM/5(VINP_SolarRErr_enum) -> [VINP_SolarRErr_enum]
  Zone_Dr_THCM/6(VINP_TFaceL_C) -> [VINP_TFaceL_C]
  Zone_Dr_THCM/7(VINP_TFaceLErr_enum) -> [VINP_TFaceLErr_enum]
  Zone_Dr_THCM/8(VINP_TFaceR_C) -> [VINP_TFaceR_C]
  Zone_Dr_THCM/9(VINP_TFaceRErr_enum) -> [VINP_TFaceRErr_enum]
  Zone_Dr_THCM/10(VINP_TFaceRr_C) -> [VINP_TFaceRr_C]
  Zone_Dr_THCM/11(VINP_TFaceRrErr_enum) -> [VINP_TFaceRrErr_enum]
  Zone_Dr_THCM/12(VINP_TFootL_C) -> [VINP_TFootL_C]
  Zone_Dr_THCM/13(VINP_TFootLErr_enum) -> [VINP_TFootLErr_enum]
  Zone_Dr_THCM/14(VINP_TFootR_C) -> [VINP_TFootR_C]
  Zone_Dr_THCM/15(VINP_TFootRErr_enum) -> [VINP_TFootRErr_enum]
  Zone_Dr_THCM/16(VINP_TFootRr_C) -> [VINP_TFootRr_C]
  Zone_Dr_THCM/17(VINP_TFootRrErr_enum) -> [VINP_TFootRrErr_enum]
  Zone_Dr_THCM/18(VINP_Tevap_C) -> [VINP_Tevap_C]
  Zone_Dr_THCM/19(VINP_TevapErr_enum) -> [VINP_TevapErr_enum]
  Zone_Dr_THCM/20(VINP_Tincar_C) -> [VINP_Tincar_C]
  Zone_Dr_THCM/21(VINP_TincarErr_enum) -> [VINP_TincarErr_enum]
  [BHAL_outputs] -> Zone_Dr_VCU/1(BHAL_outputs)
  [inp_CanValid_bus] -> Zone_Dr_VCU/2(inp_CanValid_bus)
  Zone_Dr_VCU/1(VINP_DrAuBoxPwrN1Curr_A) -> [VINP_DrAuBoxPwrN1Curr_A]
  Zone_Dr_VCU/2(VINP_DrAuBoxPwrN2Curr_A) -> [VINP_DrAuBoxPwrN2Curr_A]
  Zone_Dr_VCU/3(VINP_DrColumnSWFault_enum) -> [VINP_DrColumnSWFault_enum]
  Zone_Dr_VCU/4(VINP_DrCtrlBDVolt_V) -> [VINP_DrCtrlBDVolt_V]
  Zone_Dr_VCU/5(VINP_DrCtrlTemp_C) -> [VINP_DrCtrlTemp_C]
  Zone_Dr_VCU/6(VINP_DrEOBDFault_enum) -> [VINP_DrEOBDFault_enum]
  Zone_Dr_VCU/7(VINP_DrIVIFault_enum) -> [VINP_DrIVIFault_enum]
  Zone_Dr_VCU/8(VINP_DrInfoFault_enum) -> [VINP_DrInfoFault_enum]
  Zone_Dr_VCU/9(VINP_DrPMMLVOutPErrLmp_flg) -> [VINP_DrPMMLVOutPErrLmp_flg]
  Zone_Dr_VCU/10(VINP_DrPMMLimpHomeActReq_flg) -> [VINP_DrPMMLimpHomeActReq_flg]
  Zone_Dr_VCU/11(VINP_DrPMMSysErrLmp_flg) -> [VINP_DrPMMSysErrLmp_flg]
  Zone_Dr_VCU/12(VINP_DrPowerTemp1_C) -> [VINP_DrPowerTemp1_C]
  Zone_Dr_VCU/13(VINP_DrPowerTemp2_C) -> [VINP_DrPowerTemp2_C]
  Zone_Dr_VCU/14(VINP_DrPwrInformationSta_flg) -> [VINP_DrPwrInformationSta_flg]
  Zone_Dr_VCU/15(VINP_DrPwrONA1Curr_A) -> [VINP_DrPwrONA1Curr_A]
  Zone_Dr_VCU/16(VINP_DrPwrONA2Curr_A) -> [VINP_DrPwrONA2Curr_A]
  Zone_Dr_VCU/17(VINP_DrPwrSta_enum) -> [VINP_DrPwrSta_enum]
  Zone_Dr_VCU/18(VINP_DrPwrStdbyACurr_A) -> [VINP_DrPwrStdbyACurr_A]
  Zone_Dr_VCU/19(VINP_DrPwrWindowECUFault_enum) -> [VINP_DrPwrWindowECUFault_enum]
  Zone_Dr_VCU/20(VINP_DrStdAErrSta_flg) -> [VINP_DrStdAErrSta_flg]
  Zone_Dr_VCU/21(VINP_DrTHCMFault_enum) -> [VINP_DrTHCMFault_enum]
  Zone_Dr_VCU/22(VINP_ZoneDrMalfunLevel_enum) -> [VINP_ZoneDrMalfunLevel_enum]
  [BHAL_outputs] -> Zone_Fr_THCM/1(BHAL_outputs)
  [inp_CanValid_bus] -> Zone_Fr_THCM/2(inp_CanValid_bus)
  Zone_Fr_THCM/1(VINP_AGSErr_enum) -> [VINP_AGSErr_enum]
  Zone_Fr_THCM/2(VINP_BatInTemp_C) -> [VINP_BatInTemp_C]
  Zone_Fr_THCM/3(VINP_BatInTempErr_enum) -> [VINP_BatInTempErr_enum]
  Zone_Fr_THCM/4(VINP_BatOutTemp_C) -> [VINP_BatOutTemp_C]
  Zone_Fr_THCM/5(VINP_COMPErr_enum) -> [VINP_COMPErr_enum]
  Zone_Fr_THCM/6(VINP_EACProtectEnable_enum) -> [VINP_EACProtectEnable_enum]
  Zone_Fr_THCM/7(VINP_EWP3Err_enum) -> [VINP_EWP3Err_enum]
  Zone_Fr_THCM/8(VINP_EXV1Err_enum) -> [VINP_EXV1Err_enum]
  Zone_Fr_THCM/9(VINP_EXV2Err_enum) -> [VINP_EXV2Err_enum]
  Zone_Fr_THCM/10(VINP_FanErr_enum) -> [VINP_FanErr_enum]
  Zone_Fr_THCM/11(VINP_MotorInTemp_C) -> [VINP_MotorInTemp_C]
  Zone_Fr_THCM/12(VINP_MotorInTempErr_enum) -> [VINP_MotorInTempErr_enum]
  Zone_Fr_THCM/13(VINP_MotorOutTemp_C) -> [VINP_MotorOutTemp_C]
  Zone_Fr_THCM/14(VINP_MotorOutTempErr_enum) -> [VINP_MotorOutTempErr_enum]
  Zone_Fr_THCM/15(VINP_PTHighP_KPa) -> [VINP_PTHighP_KPa]
  Zone_Fr_THCM/16(VINP_PTHighPErr_enum) -> [VINP_PTHighPErr_enum]
  Zone_Fr_THCM/17(VINP_PTHighTact_C) -> [VINP_PTHighTact_C]
  Zone_Fr_THCM/18(VINP_PTHighTactErr_enum) -> [VINP_PTHighTactErr_enum]
  Zone_Fr_THCM/19(VINP_PTLowP1_KPa) -> [VINP_PTLowP1_KPa]
  Zone_Fr_THCM/20(VINP_PTLowP1Err_enum) -> [VINP_PTLowP1Err_enum]
  Zone_Fr_THCM/21(VINP_PTLowP2_KPa) -> [VINP_PTLowP2_KPa]
  Zone_Fr_THCM/22(VINP_PTLowP2Err_enum) -> [VINP_PTLowP2Err_enum]
  Zone_Fr_THCM/23(VINP_PTLowT1_C) -> [VINP_PTLowT1_C]
  Zone_Fr_THCM/24(VINP_PTLowT1Err_enum) -> [VINP_PTLowT1Err_enum]
  Zone_Fr_THCM/25(VINP_PTLowT2_C) -> [VINP_PTLowT2_C]
  Zone_Fr_THCM/26(VINP_PTLowT2Err_enum) -> [VINP_PTLowT2Err_enum]
  Zone_Fr_THCM/27(VINP_SOTXVErr_enum) -> [VINP_SOTXVErr_enum]
  Zone_Fr_THCM/28(VINP_SOV1Err_enum) -> [VINP_SOV1Err_enum]
  Zone_Fr_THCM/29(VINP_SOV2Err_enum) -> [VINP_SOV2Err_enum]
  Zone_Fr_THCM/30(VINP_SOV3Err_enum) -> [VINP_SOV3Err_enum]
  Zone_Fr_THCM/31(VINP_Tamb_C) -> [VINP_Tamb_C]
  Zone_Fr_THCM/32(VINP_TambErr_enum) -> [VINP_TambErr_enum]
  bus_creator/1 -> inp_Hal_bus/1
  [VINP_DKCReVehData_enum] -> bus_creator/1
  [VINP_DKCRemotePW_enum] -> bus_creator/2
  [VINP_PCommandToBCM_enum] -> bus_creator/3
  [VINP_PCommandToPTG_enum] -> bus_creator/4
  [VINP_PDKeyAreaLockUnlock_enum] -> bus_creator/5
  [VINP_PDKeyAreaPS_enum] -> bus_creator/6
  [VINP_PDKeyAreaPTG_enum] -> bus_creator/7
  [VINP_PDKeyWelcome_enum] -> bus_creator/8
  [VINP_PDkeyShowIVI_enum] -> bus_creator/9
  [VINP_PKeyMiss_flg] -> bus_creator/10
  [VINP_PKeyMode_enum] -> bus_creator/11
  [VINP_PUIDLowPower_flg] -> bus_creator/12
  [VINP_EncryptionDATA063_enum] -> bus_creator/13
  [VINP_EncryptionDATA64127_enum] -> bus_creator/14
  [VINP_RandomNumberX_enum] -> bus_creator/15
  [VINP_PTGRDILSta_enum] -> bus_creator/16
  [VINP_CSWDimSw_flg] -> bus_creator/17
  [VINP_CSWFWasSwSta_enum] -> bus_creator/18
  [VINP_CSWFWipSwSta_enum] -> bus_creator/19
  [VINP_CSWPassSWSta_flg] -> bus_creator/20
  [VINP_CSWRWasSWSta_enum] -> bus_creator/21
  [VINP_CSWRWipIntSwSta_enum] -> bus_creator/22
  [VINP_CSWTurnSwSta_enum] -> bus_creator/23
  [VINP_DrLockSta_flg] -> bus_creator/24
  [VINP_MIRRORFOLDSW_flg] -> bus_creator/25
  [VINP_RLSLampSta_flg] -> bus_creator/26
  [VINP_RLSRainSnrWiperCmd_enum] -> bus_creator/27
  [VINP_RLTurnLampC_mA] -> bus_creator/28
  [VINP_RRTurnLampC_mA] -> bus_creator/29
  [VINP_RWiperAS_flg] -> bus_creator/30
  [VINP_RWiperProtection_flg] -> bus_creator/31
  [VINP_SWCCANCELSta_flg] -> bus_creator/32
  [VINP_SWCResUpSta_flg] -> bus_creator/33
  [VINP_SWCSetdownSta_flg] -> bus_creator/34
  [VINP_SWCmodeSta_flg] -> bus_creator/35
  [VINP_LDrvValWdwOpened_pct] -> bus_creator/36
  [VINP_LPasValWdwOpened_pct] -> bus_creator/37
  [VINP_LRLDValWdwOpened_pct] -> bus_creator/38
  [VINP_LRRDValWdwOpened_pct] -> bus_creator/39
  [VINP_PTGInnerSW2_enum] -> bus_creator/40
  [VINP_FrntPTCRearLeActHeatPwr_W] -> bus_creator/41
  [VINP_FrntPTCRearRiActHeatPwr_W] -> bus_creator/42
  [VINP_FrntPTCRiActHeatPwr_W] -> bus_creator/43
  [VINP_FLTurnLampC_mA] -> bus_creator/44
  [VINP_FRTurnLampC_mA] -> bus_creator/45
  [VINP_FWiperAS_flg] -> bus_creator/46
  [VINP_FWiperProtection_flg] -> bus_creator/47
  [VINP_COMPStatorSpd_rpm] -> bus_creator/48
  [VINP_CompProEN_flg] -> bus_creator/49
  [VINP_DrSCPSysErrLmp_flg] -> bus_creator/50
  [VINP_RegenMode_enum] -> bus_creator/51
  [VINP_SetSpd_kph] -> bus_creator/52
  [VINP_ZoneSpdCtrlMode_enum] -> bus_creator/53
  [VINP_BlowerErr_enum] -> bus_creator/54
  [VINP_SolarL_W] -> bus_creator/55
  [VINP_SolarLErr_enum] -> bus_creator/56
  [VINP_SolarR_W] -> bus_creator/57
  [VINP_SolarRErr_enum] -> bus_creator/58
  [VINP_TFaceL_C] -> bus_creator/59
  [VINP_TFaceLErr_enum] -> bus_creator/60
  [VINP_TFaceR_C] -> bus_creator/61
  [VINP_TFaceRErr_enum] -> bus_creator/62
  [VINP_TFaceRr_C] -> bus_creator/63
  [VINP_TFaceRrErr_enum] -> bus_creator/64
  [VINP_TFootL_C] -> bus_creator/65
  [VINP_TFootLErr_enum] -> bus_creator/66
  [VINP_TFootR_C] -> bus_creator/67
  [VINP_TFootRErr_enum] -> bus_creator/68
  [VINP_TFootRr_C] -> bus_creator/69
  [VINP_TFootRrErr_enum] -> bus_creator/70
  [VINP_Tevap_C] -> bus_creator/71
  [VINP_TevapErr_enum] -> bus_creator/72
  [VINP_Tincar_C] -> bus_creator/73
  [VINP_TincarErr_enum] -> bus_creator/74
  [VINP_DrAuBoxPwrN1Curr_A] -> bus_creator/75
  [VINP_DrAuBoxPwrN2Curr_A] -> bus_creator/76
  [VINP_DrColumnSWFault_enum] -> bus_creator/77
  [VINP_DrCtrlBDVolt_V] -> bus_creator/78
  [VINP_DrCtrlTemp_C] -> bus_creator/79
  [VINP_DrEOBDFault_enum] -> bus_creator/80
  [VINP_DrIVIFault_enum] -> bus_creator/81
  [VINP_DrInfoFault_enum] -> bus_creator/82
  [VINP_DrPMMLVOutPErrLmp_flg] -> bus_creator/83
  [VINP_DrPMMLimpHomeActReq_flg] -> bus_creator/84
  [VINP_DrPMMSysErrLmp_flg] -> bus_creator/85
  [VINP_DrPowerTemp1_C] -> bus_creator/86
  [VINP_DrPowerTemp2_C] -> bus_creator/87
  [VINP_DrPwrInformationSta_flg] -> bus_creator/88
  [VINP_DrPwrONA1Curr_A] -> bus_creator/89
  [VINP_DrPwrONA2Curr_A] -> bus_creator/90
  [VINP_DrPwrSta_enum] -> bus_creator/91
  [VINP_DrPwrStdbyACurr_A] -> bus_creator/92
  [VINP_DrPwrWindowECUFault_enum] -> bus_creator/93
  [VINP_DrStdAErrSta_flg] -> bus_creator/94
  [VINP_DrTHCMFault_enum] -> bus_creator/95
  [VINP_ZoneDrMalfunLevel_enum] -> bus_creator/96
  [VINP_AGSErr_enum] -> bus_creator/97
  [VINP_BatInTemp_C] -> bus_creator/98
  [VINP_BatInTempErr_enum] -> bus_creator/99
  [VINP_BatOutTemp_C] -> bus_creator/100
  [VINP_COMPErr_enum] -> bus_creator/101
  [VINP_EACProtectEnable_enum] -> bus_creator/102
  [VINP_EWP3Err_enum] -> bus_creator/103
  [VINP_EXV1Err_enum] -> bus_creator/104
  [VINP_EXV2Err_enum] -> bus_creator/105
  [VINP_FanErr_enum] -> bus_creator/106
  [VINP_MotorInTemp_C] -> bus_creator/107
  [VINP_MotorInTempErr_enum] -> bus_creator/108
  [VINP_MotorOutTemp_C] -> bus_creator/109
  [VINP_MotorOutTempErr_enum] -> bus_creator/110
  [VINP_PTHighP_KPa] -> bus_creator/111
  [VINP_PTHighPErr_enum] -> bus_creator/112
  [VINP_PTHighTact_C] -> bus_creator/113
  [VINP_PTHighTactErr_enum] -> bus_creator/114
  [VINP_PTLowP1_KPa] -> bus_creator/115
  [VINP_PTLowP1Err_enum] -> bus_creator/116
  [VINP_PTLowP2_KPa] -> bus_creator/117
  [VINP_PTLowP2Err_enum] -> bus_creator/118
  [VINP_PTLowT1_C] -> bus_creator/119
  [VINP_PTLowT1Err_enum] -> bus_creator/120
  [VINP_PTLowT2_C] -> bus_creator/121
  [VINP_PTLowT2Err_enum] -> bus_creator/122
  [VINP_SOTXVErr_enum] -> bus_creator/123
  [VINP_SOV1Err_enum] -> bus_creator/124
  [VINP_SOV2Err_enum] -> bus_creator/125
  [VINP_SOV3Err_enum] -> bus_creator/126
  [VINP_Tamb_C] -> bus_creator/127
  [VINP_TambErr_enum] -> bus_creator/128

== system inp/INP/CAN5/CommunicationCheck ==
  BHAL_outputs : Inport
  CANMsgInvalidTBOX1 : FVT_lib/inp/CAN_Msg_Validity_Process_template  SystemSampleTime=-1  VariantActivationTime=update diagram  Latency=0  AutoFrameSizeCalculation=off
      link override debdec: Value=KINP_CANMsgInvalidTBOX1_flg_debdec
      link override debinc: Value=KINP_CANMsgInvalidTBOX1_flg_debinc
      link override deblim: Value=KINP_CANMsgInvalidTBOX1_flg_deblim
      link override inverse: Value=KINP_CANMsgInvalidTBOX1_flg_inverse
      link override ovrdflg: Value=KINP_CANMsgInvalidTBOX1_flg_ovrdflg
      link override ovrdval: Value=KINP_CANMsgInvalidTBOX1_flg_ovrdval
      link override srvcflg: Value=KINP_CANMsgInvalidTBOX1_flg_srvcflg
      link override srvcval: Value=KINP_CANMsgInvalidTBOX1_flg_srvcval
  bus_creator : BusCreator  Inputs=1
  bus_selector : BusSelector  OutputSignals=VHAL_CANMsgInvalidTBOX1_flg
  not1 : Logic  Operator=NOT  AllPortsSameDT=off  OutDataTypeStr=boolean
  inp_CanValid_bus : Outport
  wires:
  BHAL_outputs/1 -> [BHAL_outputs]
  bus_selector/1 -> CANMsgInvalidTBOX1/1  "<VHAL_CANMsgInvalidTBOX1_flg>"
  CANMsgInvalidTBOX1/1 -> not1/1
  not1/1 -> bus_creator/1  "VINP_CANMsgValidTBOX1_flg"
  [BHAL_outputs] -> bus_selector/1
  bus_creator/1 -> inp_CanValid_bus/1

== system inp/INP/CAN5/CreateBus ==
  inp_CanValid_bus : Inport
  inp_Hal_bus : Inport  Port=2
  UnitConverter_1 : DataTypeConversion  OutDataTypeStr=boolean
  UnitConverter_2 : DataTypeConversion  OutDataTypeStr=single
  UnitConverter_3 : DataTypeConversion  OutDataTypeStr=uint8
  UnitConverter_4 : DataTypeConversion  OutDataTypeStr=uint16
  UnitConverter_5 : DataTypeConversion  OutDataTypeStr=uint8
  UnitConverter_6 : DataTypeConversion  OutDataTypeStr=single
  UnitConverter_7 : DataTypeConversion  OutDataTypeStr=boolean
  bus_creator : BusCreator  Inputs=7
  bus_selector : BusSelector  OutputSignals=VINP_CANMsgValidTBOX1_flg
  bus_selector_1 : BusSelector  OutputSignals=VINP_PowerOffTSet_cnt,VINP_ReOutsideMirror_enum,VINP_ReDoorLock_enum,VINP_RePwrReqTbox_enum,VINP_RemoteACTemp_C,VINP_RemoteAutoReq_flg
  BINP_outputs : Outport
  wires:
  inp_CanValid_bus/1 -> [inp_CanValid_bus]
  inp_Hal_bus/1 -> [inp_Hal_bus]
  bus_selector/1 -> UnitConverter_1/1  "<VINP_CANMsgValidTBOX1_flg>"
  UnitConverter_1/1 -> bus_creator/1  "VINP_CANMsgValidTBOX1_flg"
  bus_selector_1/1 -> UnitConverter_2/1  "<VINP_PowerOffTSet_cnt>"
  UnitConverter_2/1 -> bus_creator/2  "VINP_PowerOffTSet_cnt"
  bus_selector_1/2 -> UnitConverter_3/1  "<VINP_ReOutsideMirror_enum>"
  UnitConverter_3/1 -> bus_creator/3  "VINP_ReOutsideMirror_enum"
  bus_selector_1/3 -> UnitConverter_4/1  "<VINP_ReDoorLock_enum>"
  UnitConverter_4/1 -> bus_creator/4  "VINP_ReDoorLock_enum"
  bus_selector_1/4 -> UnitConverter_5/1  "<VINP_RePwrReqTbox_enum>"
  UnitConverter_5/1 -> bus_creator/5  "VINP_RePwrReqTbox_enum"
  bus_selector_1/5 -> UnitConverter_6/1  "<VINP_RemoteACTemp_C>"
  UnitConverter_6/1 -> bus_creator/6  "VINP_RemoteACTemp_C"
  bus_selector_1/6 -> UnitConverter_7/1  "<VINP_RemoteAutoReq_flg>"
  UnitConverter_7/1 -> bus_creator/7  "VINP_RemoteAutoReq_flg"
  [inp_CanValid_bus] -> bus_selector/1
  [inp_Hal_bus] -> bus_selector_1/1
  bus_creator/1 -> BINP_outputs/1

== system inp/INP/CAN5/SignalCheck ==
  inp_CanValid_bus : Inport
  TASK_TIME_S : Inport  Port=2
  BHAL_outputs : Inport  Port=3
  TBOX1 : Subsystem
  bus_creator : BusCreator  Inputs=6
  inp_Hal_bus : Outport
  wires:
  inp_CanValid_bus/1 -> [inp_CanValid_bus]
  TASK_TIME_S/1 -> [TASK_TIME_S]
  BHAL_outputs/1 -> [BHAL_outputs]
  [BHAL_outputs] -> TBOX1/1(BHAL_outputs)
  [inp_CanValid_bus] -> TBOX1/2(inp_CanValid_bus)
  TBOX1/1(VINP_PowerOffTSet_cnt) -> [VINP_PowerOffTSet_cnt]
  TBOX1/2(VINP_ReOutsideMirror_enum) -> [VINP_ReOutsideMirror_enum]
  TBOX1/3(VINP_ReDoorLock_enum) -> [VINP_ReDoorLock_enum]
  TBOX1/4(VINP_RePwrReqTbox_enum) -> [VINP_RePwrReqTbox_enum]
  TBOX1/5(VINP_RemoteACTemp_C) -> [VINP_RemoteACTemp_C]
  TBOX1/6(VINP_RemoteAutoReq_flg) -> [VINP_RemoteAutoReq_flg]
  bus_creator/1 -> inp_Hal_bus/1
  [VINP_PowerOffTSet_cnt] -> bus_creator/1
  [VINP_ReOutsideMirror_enum] -> bus_creator/2
  [VINP_ReDoorLock_enum] -> bus_creator/3
  [VINP_RePwrReqTbox_enum] -> bus_creator/4
  [VINP_RemoteACTemp_C] -> bus_creator/5
  [VINP_RemoteAutoReq_flg] -> bus_creator/6

== system inp/INP/GPIO/Analog ==
  BHAL_outputs : Inport
  TASK_TIME_S : Inport  Port=2
  AccelPedal1Vol_V : FVT_lib/inp/ad_signal_template  SystemSampleTime=-1  VariantActivationTime=update diagram  Latency=0  AutoFrameSizeCalculation=off
      link override defval: Value=KINP_AccelPedal1Vol_V_defval
      link override fftdec: Value=KINP_AccelPedal1Vol_V_fftdec
      link override fftinc: Value=KINP_AccelPedal1Vol_V_fftinc
      link override fftlim: Value=KINP_AccelPedal1Vol_V_fftlim
      link override limlow: Value=KINP_AccelPedal1Vol_V_limlow
      link override limupr: Value=KINP_AccelPedal1Vol_V_limupr
      link override ovrdflg: Value=KINP_AccelPedal1Vol_V_ovrdflg
      link override ovrdval: Value=KINP_AccelPedal1Vol_V_ovrdval
      link override srvcflg: Value=KINP_AccelPedal1Vol_V_srvcflg
      link override srvcval: Value=KINP_AccelPedal1Vol_V_srvcval
      link override tcfilt: Value=KINP_AccelPedal1Vol_V_tcfilt
  AccelPedal2Vol_V : FVT_lib/inp/ad_signal_template  SystemSampleTime=-1  VariantActivationTime=update diagram  Latency=0  AutoFrameSizeCalculation=off
      link override defval: Value=KINP_AccelPedal2Vol_V_defval
      link override fftdec: Value=KINP_AccelPedal2Vol_V_fftdec
      link override fftinc: Value=KINP_AccelPedal2Vol_V_fftinc
      link override fftlim: Value=KINP_AccelPedal2Vol_V_fftlim
      link override limlow: Value=KINP_AccelPedal2Vol_V_limlow
      link override limupr: Value=KINP_AccelPedal2Vol_V_limupr
      link override ovrdflg: Value=KINP_AccelPedal2Vol_V_ovrdflg
      link override ovrdval: Value=KINP_AccelPedal2Vol_V_ovrdval
      link override srvcflg: Value=KINP_AccelPedal2Vol_V_srvcflg
      link override srvcval: Value=KINP_AccelPedal2Vol_V_srvcval
      link override tcfilt: Value=KINP_AccelPedal2Vol_V_tcfilt
  Bus Selector : BusSelector  OutputSignals=VHAL_AccelPedal1Vol_V
  Bus Selector1 : BusSelector  OutputSignals=VHAL_AccelPedal2Vol_V
  Constant{,1..3} (4 alike) : Constant  Value=FALSE
  VINP_AccelPedal1VolShortHigh_enum : Outport
  VINP_AccelPedal1VolShortLow_enum : Outport  Port=2
  VINP_AccelPedal1Vol_V : Outport  Port=3
  VINP_AccelPedal1VolValid_flg : Outport  Port=4
  VINP_AccelPedal2VolShortHigh_enum : Outport  Port=5
  VINP_AccelPedal2VolShortLow_enum : Outport  Port=6
  VINP_AccelPedal2Vol_V : Outport  Port=7
  VINP_AccelPedal2VolValid_flg : Outport  Port=8
  wires:
  BHAL_outputs/1 -> [BHAL_outputs]
  TASK_TIME_S/1 -> [TASK_TIME_S]
  AccelPedal1Vol_V/1 -> VINP_AccelPedal1VolShortHigh_enum/1  "VINP_AccelPedal1VolShortHigh_enum"
  AccelPedal1Vol_V/2 -> VINP_AccelPedal1VolShortLow_enum/1  "VINP_AccelPedal1VolShortLow_enum"
  AccelPedal1Vol_V/3 -> VINP_AccelPedal1Vol_V/1  "VINP_AccelPedal1Vol_V"
  AccelPedal1Vol_V/4 -> VINP_AccelPedal1VolValid_flg/1  "VINP_AccelPedal1VolValid_flg"
  AccelPedal2Vol_V/1 -> VINP_AccelPedal2VolShortHigh_enum/1  "VINP_AccelPedal2VolShortHigh_enum"
  AccelPedal2Vol_V/2 -> VINP_AccelPedal2VolShortLow_enum/1  "VINP_AccelPedal2VolShortLow_enum"
  AccelPedal2Vol_V/3 -> VINP_AccelPedal2Vol_V/1  "VINP_AccelPedal2Vol_V"
  AccelPedal2Vol_V/4 -> VINP_AccelPedal2VolValid_flg/1  "VINP_AccelPedal2VolValid_flg"
  [TASK_TIME_S] -> AccelPedal1Vol_V/4
  Constant1/1 -> AccelPedal1Vol_V/3
  Constant/1 -> AccelPedal1Vol_V/2
  [BHAL_outputs] -> Bus Selector/1
  Bus Selector/1 -> AccelPedal1Vol_V/1  "<VHAL_AccelPedal1Vol_V>"
  Bus Selector1/1 -> AccelPedal2Vol_V/1  "<VHAL_AccelPedal2Vol_V>"
  [BHAL_outputs] -> Bus Selector1/1
  Constant2/1 -> AccelPedal2Vol_V/2
  Constant3/1 -> AccelPedal2Vol_V/3
  [TASK_TIME_S] -> AccelPedal2Vol_V/4
